simulink model "UUV_animation"  (Simulink 8.3)
settings: Solver=ode45  StartTime=0.0  StopTime=200  RelTol=1e-3
undefined symbols (not defined in the file or in its folder): drawUUV, P
settings Model: Creator=beard  LastModifiedBy=jhl48
settings OptimizationCC: ExpressionDepthLimit=2147483647  InitFltsAndDblsToZero=on
settings DebuggingCC: FcnCallInpInsideContextMsg=UseLocalSettings

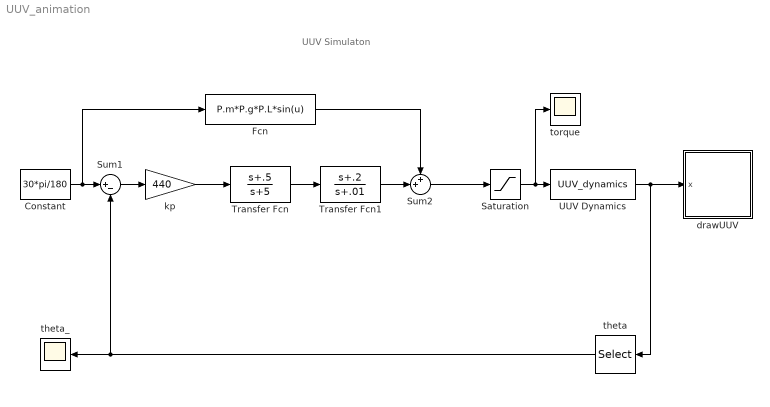
== system UUV_animation ==
  note: UUV Simulaton
  Constant : Constant  Value=30*pi/180
  Fcn : Fcn  Expr=P.m*P.g*P.L*sin(u)
  Saturation : Saturate  UpperLimit=250  LowerLimit=-250
  Sum1 : Sum  Inputs=|+-
  Sum2 : Sum  Inputs=++|
  Transfer Fcn : TransferFcn  Numerator=[1 .5]  Denominator=[1 5]
  Transfer Fcn1 : TransferFcn  Numerator=[1 .2]  Denominator=[1 .01]
  UUV Dynamics : S-Function  FunctionName=UUV_dynamics  Parameters=P  EnableBusSupport=off
  drawUUV : Subsystem
      mask init:
      | % drawing parameters
      | L = 1;
      | w = 0.3;
      | 
      | MajorAxis = 10;
      | MinorAxis = 6;
      | C_M = [0;-4];
      mask Display: image(imread('tv.jpg'))
  kp : Gain  Gain=440
  theta : Selector  InputPortWidth=2  Indices=[1]
  theta_ : Scope
      settings: TimeRange=100  YMin=0.497419  YMax=0.549779
  torque : Scope
      settings: TimeRange=1000  YMin=-50  YMax=250
  wires:
  UUV Dynamics/1 -> drawUUV/1(x), theta/1
  Saturation/1 -> UUV Dynamics/1, torque/1
  Transfer Fcn/1 -> Transfer Fcn1/1
  Sum1/1 -> kp/1
  Constant/1 -> Fcn/1, Sum1/1
  theta/1 -> theta_/1, Sum1/2
  kp/1 -> Transfer Fcn/1
  Fcn/1 -> Sum2/1
  Transfer Fcn1/1 -> Sum2/2
  Sum2/1 -> Saturation/1

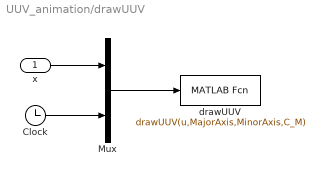
== system UUV_animation/drawUUV ==
  x : Inport
  Clock : Clock
  Mux : Mux  Inputs=2
  "drawUUV " : MATLABFcn  MATLABFcn=drawUUV(u,MajorAxis,MinorAxis,C_M)  OutputDimensions=0  SampleTime=0.1
  wires:
  Mux/1 -> "drawUUV "/1
  x/1 -> Mux/1
  Clock/1 -> Mux/2
